simulink model "CalcSys"  (R2016a)
settings: Solver=FixedStepDiscrete  StartTime=0.0  StopTime=10.0  RelTol=1e-3
settings Model: Creator=WINDOWS  LastModifiedBy=WINDOWS
settings OptimizationCC: DefaultParameterBehavior=Inlined  InlineInvariantSignals=on  EnableMemcpy=off  OptimizeModelRefInitCode=on  LifeSpan=1
settings DebuggingCC: UnderspecifiedInitializationDetection=Classic  MergeDetectMultiDrivingBlocksExec=none  StrictBusMsg=Warning
settings ModelReferenceCC: PropagateSignalLabelsOutOfModel=off
settings RTWCC: SystemTargetFile=ert.tlc  GenCodeOnly=on  TemplateMakefile=ert_default_tmf  GenerateReport=on  IncludeHyperlinkInReport=on  LaunchReport=on  GenerateTraceInfo=on  GenerateTraceReport=on  GenerateTraceReportSl=on  GenerateTraceReportSf=on  GenerateTraceReportEml=on
settings CodeAppCC: ForceParamTrailComments=on  IgnoreCustomStorageClasses=off  OperatorAnnotations=on  SimulinkDataObjDesc=on  SFDataObjDesc=on  MATLABFcnDesc=on  InsertBlockDesc=on  MATLABSourceComments=on
settings ERTTargetCC: GenerateSampleERTMain=on  InlinedParameterPlacement=NonHierarchical  ERTCustomFileTemplate=example_file_process.tlc

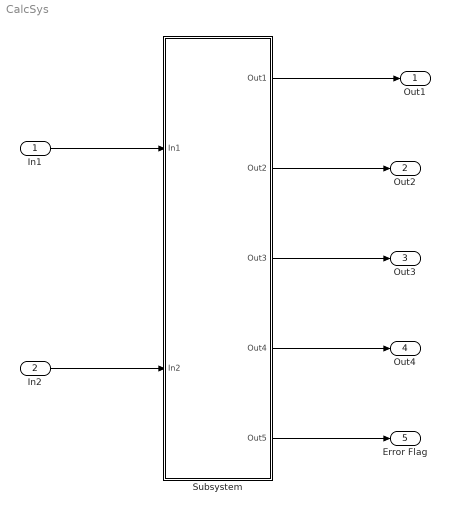
== system CalcSys ==
  In1 : Inport
  In2 : Inport  Port=2
  Subsystem : Subsystem
  Out1 : Outport
  Out2 : Outport  Port=2
  Out3 : Outport  Port=3
  Out4 : Outport  Port=4
  Error Flag : Outport  Port=5
  wires:
  In1/1 -> Subsystem/1(In1)
  In2/1 -> Subsystem/2(In2)
  Subsystem/1(Out1) -> Out1/1
  Subsystem/2(Out2) -> Out2/1
  Subsystem/3(Out3) -> Out3/1
  Subsystem/4(Out4) -> Out4/1
  Subsystem/5(Out5) -> Error Flag/1

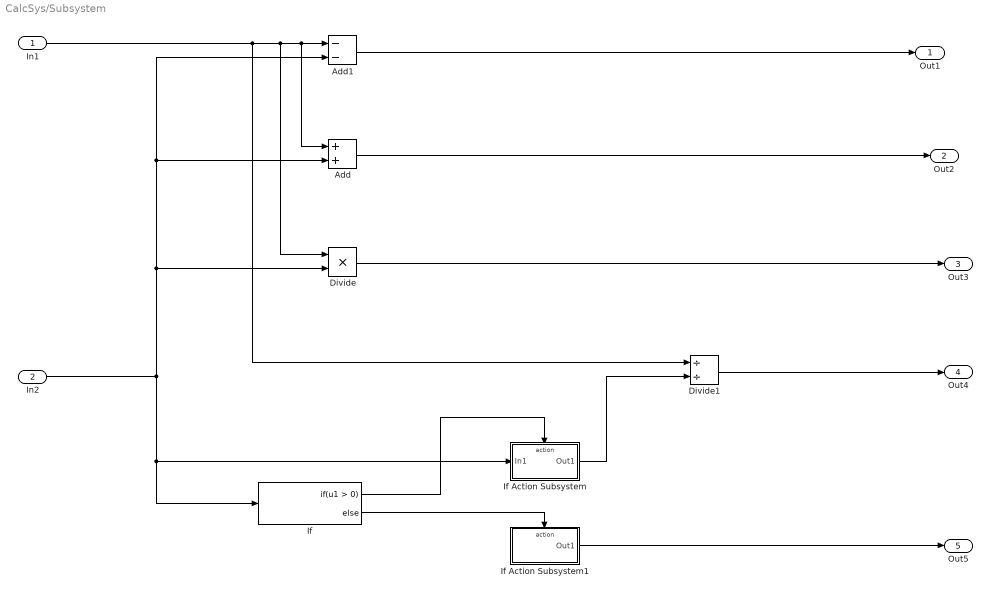
== system CalcSys/Subsystem ==
  In1 : Inport
  In2 : Inport  Port=2
  Add : Sum
  Add1 : Sum  Inputs=--
  Divide : Product  Inputs=**
  Divide1 : Product  Inputs=//
  If : If
  If Action Subsystem : Subsystem  TreatAsAtomicUnit=on
  If Action Subsystem1 : Subsystem  TreatAsAtomicUnit=on
  Out1 : Outport
  Out2 : Outport  Port=2
  Out3 : Outport  Port=3
  Out4 : Outport  Port=4
  Out5 : Outport  Port=5
  wires:
  If Action Subsystem/1(Out1) -> Divide1/2
  Add/1 -> Out2/1
  If/1 -> If Action Subsystem/Action
  In2/1 -> Add1/2, Add/2, Divide/2, If/1, If Action Subsystem/1(In1)
  If Action Subsystem1/1(Out1) -> Out5/1
  In1/1 -> Add1/1, Add/1, Divide/1, Divide1/1
  Divide1/1 -> Out4/1
  If/2 -> If Action Subsystem1/Action
  Add1/1 -> Out1/1
  Divide/1 -> Out3/1

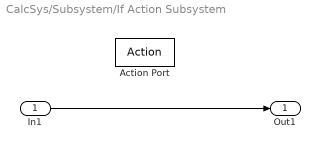
== system CalcSys/Subsystem/If Action Subsystem ==
  In1 : Inport
  Action Port : ActionPort  ActionType=then
  Out1 : Outport
  wires:
  In1/1 -> Out1/1

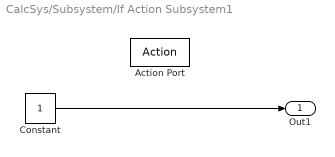
== system CalcSys/Subsystem/If Action Subsystem1 ==
  Action Port : ActionPort  ActionType=else
  Constant : Constant
  Out1 : Outport
  wires:
  Constant/1 -> Out1/1
